simulink model "PubIfDecisionTOS_MDL"  (R2020b)
settings: configuration reference "DspaceConfig" (kept outside this file)
PostLoadFcn:
  | if any(exist('dsrtsu_mdlpostloadfcn', 'file') ~= 0), dsrtsu_mdlpostloadfcn('Execute', bdroot); end
InitFcn:
  | , if any(exist('dsmpb_private', 'file') ~= 0), dsmpb_private('dsmpb_mdlclblib', 'Init', bdroot); end,
undefined symbols (not defined in the file or in its folder): C_TOS_ACCEgoRAxletoFbumplength_m, C_TOS_ACCTargetFront_Flag, C_TOS_AEBJAPedObjDxThre_Val, C_TOS_AEBJAPedObjDyThre_Val, C_TOS_AEBJATargetSize_Val, C_TOS_AEBJAVehObjDxThre_Val, C_TOS_AEBJAVehObjDyThre_Val, C_TOS_AEBJuncPedTargetSize_Val, C_TOS_AEBLatObjDxThre_Val, C_TOS_AEBLatPedDyThre_Val, C_TOS_AEBLatTargetSize_Val, C_TOS_AEBLongTargetInEgoFront_Flag, C_TOS_axAbsGround_Parameter, C_TOS_CameraConfirmedFlag, C_TOS_CNsubjWidth, C_TOS_CurrentLaneCoreMinWidth_Val, C_TOS_CutInProb_Val_Zero, C_TOS_CutOutProb_Val_Zero, C_TOS_D2R_Val, C_TOS_DefaultValueObjectToCenterLine_dy, C_TOS_EgoCarWidth_Val, C_TOS_EgoDxRefPoint_m, C_TOS_EgoRAxletoFbumplength_m, C_TOS_HalfWidthVehicle_Con, C_TOS_HWA_CurrentLaneFlag, C_TOS_HWA_LeftLaneFlag, C_TOS_HWA_MovingDir_Vaild, C_TOS_HWA_MovState_Vaild, C_TOS_HWA_RightLaneFlag, C_TOS_LaneLineCourseErrorFront, C_TOS_LaneLineCourseErrorRear, C_TOS_MotorbikeDefaultWidth_m, C_TOS_NumberOfEffectiveTargets, C_TOS_Obj_Age_Val, C_TOS_Objdx_Constraint_Val, C_TOS_ObjectDefaultWidth_m, C_TOS_ObjInCurrentLane_Val, C_TOS_ObjInCurrentLaneValid, C_TOS_ObjInLeftLaneValid, C_TOS_ObjInRightLaneValid, C_TOS_ObjNotInCurrentLane_Val, C_TOS_ObjNotREElementType, C_TOS_ObjPredictDis_dy_ConstantVal_Zeros, C_TOS_ObjToCenterLine_ConstantVal_Zeros, C_TOS_OFMObjIDInvilad_Val, C_TOS_PIL_LatDisCons_Val_zero, C_TOS_PIL_ObjectCutInFlag_b, C_TOS_PIL_ObjectCutOutFlag_b, C_TOS_PIL_ObjLaneProb_al_Val, C_TOS_PP_ObjFusType_FC_Confirm_b, C_TOS_PP_ObjFusType_FC_FR_Confirm_b, C_TOS_PP_ObjFusType_FR_Confirm_b, C_TOS_RE_80BoolDefault_Val, C_TOS_RE_80Single181Default_Val, C_TOS_RE_80Single255Default_Val, C_TOS_RE_80Uint8Default_Val, C_TOS_RE_D2R, C_TOS_RE_D_180_Val, C_TOS_RE_InvalidObjectID_Val, C_TOS_RE_InvalidTargetChainDir_Val ... (+142)
libraries: simulink x1650, TOS_LIB x361, canfdmsglib x14
(part 38 of 69)

== system PubIfDecisionTOS_MDL/TOS_20201112/TOS_2012080320/TOS/AEB/TOS_AEBJunct_20201208/AEBJunc_Object_Condition1/AEBJA_TargetCondition/TOS_AEBJunc_TargetsCondition/AEBJunc_VehTargetCondition ==
  note: 过滤静止目标
  Object_ID : Inport
  PP_ObjFusType_FC_FR_Confirm : Inport  Port=2
  PP_ObjFusType_FR_Confirm : Inport  Port=3
  ObjectType : Inport  Port=4
  Object_Dx : Inport  Port=5
  Object_Dy : Inport  Port=6
  PP_ObjMovingDirSignalProcessing : Inport  Port=7
  Object_HeadingAngle : Inport  Port=8
  Object_VX : Inport  Port=9
  Object_VY : Inport  Port=10
  VIE_EgoVelocity : Inport  Port=11
  psiDtOpt : Inport  Port=12
  axvRefMs2 : Inport  Port=13
  AEBJunc_VehTarget_ObjectID_K1 : Inport  Port=14
  AEBJunc_Target_ObjectType_K1 : Inport  Port=15
  Object_MovingState : Inport  Port=16
  AEBJunc_VehTargetADxDyArea : Subsystem
  AEBJunc_VehTargetFusionTypeJudge : Subsystem
  AEBJunc_VehTargetObjectTypeFlag : Subsystem
  Chart : Stateflow chart  TreatAsAtomicUnit=on
  Compare To Constant : simulink/Logic and Bit Operations/Compare To Constant  relop===  const=true  OutDataTypeStr=boolean
  Logical Operator : Logic  Inputs=5  AllPortsSameDT=off  OutDataTypeStr=boolean
  Subsystem : Subsystem
  TOS_AEBJunc_VehTargetMoveDir : Subsystem
  Terminator : Terminator
  TOS_AEBJunc_VehTargetsDx : Outport
  AEBJunc_VehTargetFusionType_observal : Outport  Port=2
  AEBJunc_VehTargetObjectType_observal : Outport  Port=3
  AEBJunc_VehTargetDXDY_observal : Outport  Port=4
  AEBJunc_VehTargetMovDir_observal : Outport  Port=5
  AEBJunc_VehTargetMovState_observal : Outport  Port=6
  wires:
  [Object_ID] -> Chart/2(Object_ID)
  [AEBJunc_VehTarget_ObjectID_K1] -> Chart/4(AEBJunc_Target_ObjectID_K1)
  AEBJunc_VehTarget_ObjectID_K1/1 -> AEBJunc_VehTargetObjectTypeFlag/2(AEBJunc_VehTarget_ID_K1), [AEBJunc_VehTarget_ObjectID_K1]
  Object_ID/1 -> AEBJunc_VehTargetObjectTypeFlag/3(ObjectID), [Object_ID]
  [TOS_AEBJuncVehMovStateFlg] -> AEBJunc_VehTargetMovState_observal/1
  Subsystem/1(TOS_AEBJuncVehTargetMovStateFlg) -> [TOS_AEBJuncVehMovStateFlg], Logical Operator/5
  Object_MovingState/1 -> Subsystem/1(Object_MovingState)
  TOS_AEBJunc_VehTargetMoveDir/1(TOS_AEBJuncVehTargetMovDirFlg) -> [TOS_AEBJuncVehMovDirFlg], Logical Operator/4  "TOS_AEBJunc_VehTargetMovDir"
  Object_HeadingAngle/1 -> TOS_AEBJunc_VehTargetMoveDir/3(Object_HeadingAngle)
  PP_ObjFusType_FC_FR_Confirm/1 -> AEBJunc_VehTargetFusionTypeJudge/1(PP_ObjFusType_FC_FR_Confirm)
  [Object_Dx] -> TOS_AEBJunc_VehTargetMoveDir/1(Object_Dx)  "Object_Dx"
  [Object_Dx] -> Chart/6(Object_Dx)
  Object_Dx/1 -> [Object_Dx], AEBJunc_VehTargetADxDyArea/1(Object_Dx)
  [AEBJunc_VehFusionTypeFlag] -> AEBJunc_VehTargetFusionType_observal/1
  AEBJunc_VehTargetADxDyArea/1(TOS_AEBJunc_VehDxDyAreaFlag) -> Logical Operator/3, [TOS_AEBJunc_VehDxDyAreaFlag]
  Logical Operator/1 -> Compare To Constant/1
  Chart/1(TOS_AEBJunc_TargetsDx) -> TOS_AEBJunc_VehTargetsDx/1
  [AEBJunc_VehObjectTypeFlag] -> AEBJunc_VehTargetObjectType_observal/1
  PP_ObjMovingDirSignalProcessing/1 -> TOS_AEBJunc_VehTargetMoveDir/2(PP_ObjMovingDirSignalProcessing)
  psiDtOpt/1 -> Chart/3(psiDtOpt)
  PP_ObjFusType_FR_Confirm/1 -> AEBJunc_VehTargetFusionTypeJudge/2(PP_ObjFusType_FR_Confirm)
  Object_VY/1 -> [Object_Vy], TOS_AEBJunc_VehTargetMoveDir/5(Object_VY)
  VIE_EgoVelocity/1 -> TOS_AEBJunc_VehTargetMoveDir/6(VIE_EgoVelocity)
  AEBJunc_VehTargetFusionTypeJudge/1(AEBJunc_VehTargetFusionTypeFlag) -> [AEBJunc_VehFusionTypeFlag], Logical Operator/1
  Object_VX/1 -> TOS_AEBJunc_VehTargetMoveDir/4(Object_VX)
  Object_Dy/1 -> AEBJunc_VehTargetADxDyArea/2(Object_Dy)
  AEBJunc_VehTargetObjectTypeFlag/1(AEBJunc_VehTargetObjectTypeFlag) -> [AEBJunc_VehObjectTypeFlag], Logical Operator/2
  [TOS_AEBJuncVehMovDirFlg] -> AEBJunc_VehTargetMovDir_observal/1
  axvRefMs2/1 -> TOS_AEBJunc_VehTargetMoveDir/7(axvRefMs2)
  ObjectType/1 -> AEBJunc_VehTargetObjectTypeFlag/1(ObjectType)
  [TOS_AEBJunc_VehDxDyAreaFlag] -> AEBJunc_VehTargetDXDY_observal/1
  [Object_Vy] -> Chart/5(Object_Vy)
  Compare To Constant/1 -> Chart/1(AEBJunc_TargetCondition)
  AEBJunc_Target_ObjectType_K1/1 -> Terminator/1

== system PubIfDecisionTOS_MDL/TOS_20201112/TOS_2012080320/TOS/AEB/TOS_AEBLatCro1105/AEBLat_Object_Condition/AEBLat_TargetCondition/TOS_AEBLat_TargetsDx/AEBLat_TargetADxDyArea ==
  Object_Dx : Inport
  Object_Dy : Inport  Port=2
  Abs : Abs
  Compare To Constant1 : simulink/Logic and Bit Operations/Compare To Constant  relop=<=  const=C_TOS_AEBLatObjDxThre_Val  OutDataTypeStr=boolean
      settings: AttributesFormatString=C_TOS_AEBLatObjDxThre_Val = 40
  Compare To Constant2 : simulink/Logic and Bit Operations/Compare To Constant  relop=>  const=C_TOS_EgoDxRefPoint_m  OutDataTypeStr=boolean
      settings: AttributesFormatString=C_TOS_EgoDxRefPoint_m = 0
  Compare To Constant6 : simulink/Logic and Bit Operations/Compare To Constant  relop=<=  const=C_TOS_AEBLatPedDyThre_Val  OutDataTypeStr=boolean
      settings: AttributesFormatString=C_TOS_AEBLatPedDyThre_Val = 8 m
  Logical Operator : Logic  AllPortsSameDT=off  OutDataTypeStr=boolean
  Logical Operator1 : Logic  AllPortsSameDT=off  OutDataTypeStr=boolean
  TOS_AEBLat_DxDyAreaFlag : Outport
  wires:
  Logical Operator/1 -> Logical Operator1/1
  Object_Dy/1 -> Abs/1
  Abs/1 -> Compare To Constant6/1
  Compare To Constant1/1 -> Logical Operator/1
  Compare To Constant2/1 -> Logical Operator/2
  Logical Operator1/1 -> TOS_AEBLat_DxDyAreaFlag/1
  Compare To Constant6/1 -> Logical Operator1/2
  Object_Dx/1 -> Compare To Constant1/1, Compare To Constant2/1

== system PubIfDecisionTOS_MDL/TOS_20201112/TOS_2012080320/TOS/AEB/TOS_AEBLatCro1105/AEBLat_Object_Condition/AEBLat_TargetCondition/TOS_AEBLat_TargetsDx/AEBLat_TargetFusionTypeJudge ==
  PP_ObjFusType_FC_FR_Confirm : Inport
  PP_ObjFusType_FR_Confirm : Inport  Port=2
  Compare To Constant5 : simulink/Logic and Bit Operations/Compare To Constant  relop===  const=C_TOS_PP_ObjFusType_FC_FR_Confirm_b  OutDataTypeStr=boolean
      settings: AttributesFormatString=C_TOS_PP_ObjFusType_FC_FR_Confirm_b = 1
  Compare To Constant6 : simulink/Logic and Bit Operations/Compare To Constant  relop===  const=C_TOS_PP_ObjFusType_FR_Confirm_b  OutDataTypeStr=boolean
      settings: AttributesFormatString=C_TOS_PP_ObjFusType_FR_Confirm_b = 1
  Logical Operator : Logic  Operator=OR  AllPortsSameDT=off  OutDataTypeStr=boolean
  AEBLong_TargetFusionTypeFlag : Outport
  wires:
  PP_ObjFusType_FR_Confirm/1 -> Compare To Constant6/1
  PP_ObjFusType_FC_FR_Confirm/1 -> Compare To Constant5/1
  Compare To Constant6/1 -> Logical Operator/2
  Compare To Constant5/1 -> Logical Operator/1
  Logical Operator/1 -> AEBLong_TargetFusionTypeFlag/1

== system PubIfDecisionTOS_MDL/TOS_20201112/TOS_2012080320/TOS/AEB/TOS_AEBLatCro1105/AEBLat_Object_Condition/AEBLat_TargetCondition/TOS_AEBLat_TargetsDx/AEBLat_TargetObjectTypeFlag ==
  ObjectType : Inport
  AEBLat_Target_ID_K1 : Inport  Port=2
  ObjectID : Inport  Port=3
  AEBLat_TargetObjectTypeAborDly : Subsystem
  Compare To Constant3 : simulink/Logic and Bit Operations/Compare To Constant  relop===  const=OFM_OBJ_TYPE_E.PEDESTRIAN  OutDataTypeStr=boolean
      settings: AttributesFormatString=%<const>
  Compare To Constant4 : simulink/Logic and Bit Operations/Compare To Constant  relop===  const=OFM_OBJ_TYPE_E.MOTORBIKE  OutDataTypeStr=boolean
      settings: AttributesFormatString=%<const>
  Compare To Constant5 : simulink/Logic and Bit Operations/Compare To Constant  relop===  const=OFM_OBJ_TYPE_E.BICYCLE  OutDataTypeStr=boolean
      settings: AttributesFormatString=%<const>
  Data Type Conversion : DataTypeConversion  OutDataTypeStr=Enum: OFM_OBJ_TYPE_E
  Logical Operator3 : Logic  Operator=OR  Inputs=3  AllPortsSameDT=off  OutDataTypeStr=boolean
  AEBLat_TargetObjectTypeFlag : Outport
  wires:
  Data Type Conversion/1 -> Compare To Constant3/1, Compare To Constant4/1, Compare To Constant5/1
  ObjectType/1 -> Data Type Conversion/1
  Logical Operator3/1 -> AEBLat_TargetObjectTypeAborDly/3(TOS_AEBLat_ObjectType)
  Compare To Constant4/1 -> Logical Operator3/2
  Compare To Constant5/1 -> Logical Operator3/3
  Compare To Constant3/1 -> Logical Operator3/1
  ObjectID/1 -> AEBLat_TargetObjectTypeAborDly/2(ObjectID)
  AEBLat_Target_ID_K1/1 -> AEBLat_TargetObjectTypeAborDly/1(AEBLat_Target_ID_K1)
  AEBLat_TargetObjectTypeAborDly/1(TOS_AEBLatObjectTypeFilt) -> AEBLat_TargetObjectTypeFlag/1

== system PubIfDecisionTOS_MDL/TOS_20201112/TOS_2012080320/TOS/AEB/TOS_AEBLatCro1105/AEBLat_Object_Condition/AEBLat_TargetCondition/TOS_AEBLat_TargetsDx/TOS_AEBLat_TargetMoveDir ==
  Object_Dy : Inport
  PP_ObjMovingDirSignalProcessing : Inport  Port=2
  Object_HeadingAngle : Inport  Port=3
  Object_VX : Inport  Port=4
  Object_VY : Inport  Port=5
  VIE_EgoVelocity : Inport  Port=6
  Abs : Abs
  Abs1 : Abs
  Abs2 : Abs
  Add : Sum
  Compare To Constant : simulink/Logic and Bit Operations/Compare To Constant  relop=<  const=P_TOS_CrossingTarget_VxabsOffset_val  OutDataTypeStr=boolean
      settings: AttributesFormatString=%<const>
  Compare To Constant1 : simulink/Logic and Bit Operations/Compare To Constant  relop=>  const=P_TOS_CrossingTargetVyvThre_val  OutDataTypeStr=boolean
      settings: AttributesFormatString=%<const>
  Compare To Constant15 : simulink/Logic and Bit Operations/Compare To Constant  relop=>=  const=P_TOS_ObjLatCroYawAngMinThre_Val  OutDataTypeStr=boolean
      settings: AttributesFormatString=P_TOS_ObjLatCroYawAngMinThre_Val = 45
  Compare To Constant16 : simulink/Logic and Bit Operations/Compare To Constant  relop=<=  const=P_TOS_ObjLatCroYawAngMaxThre_Val  OutDataTypeStr=boolean
      settings: AttributesFormatString=P_TOS_ObjLatCroYawAngMaxThre_Val = 135
  Compare To Constant2 : simulink/Logic and Bit Operations/Compare To Constant  relop===  const=ObjectMovingOrientation_E.Crossing  OutDataTypeStr=boolean
      settings: AttributesFormatString=%<const>
  Data Type Conversion2 : DataTypeConversion  OutDataTypeStr=Enum: ObjectMovingOrientation_E
  Demux : Demux  Outputs=3
  Demux1 : Demux  Outputs=3
  Logical Operator : Logic  Operator=OR  Inputs=3  AllPortsSameDT=off  OutDataTypeStr=boolean
  Logical Operator{1..4,10} (5 alike) : Logic  AllPortsSameDT=off  OutDataTypeStr=boolean
  Logical Operator5 : Logic  Operator=OR  AllPortsSameDT=off  OutDataTypeStr=boolean
  Relational Operator : RelationalOperator  Operator=<  OutDataTypeStr=boolean  RndMeth=Simplest
  Relational Operator1 : RelationalOperator  Operator=<  OutDataTypeStr=boolean  RndMeth=Simplest
  Relational Operator2 : RelationalOperator  Operator=>  OutDataTypeStr=boolean  RndMeth=Simplest
  Relational Operator3 : RelationalOperator  Operator=>  OutDataTypeStr=boolean  RndMeth=Simplest
  Tapped Delay : simulink/Discrete/Tapped Delay  vinit=0.0  samptime=-1  NumDelays=2  DelayOrder=Oldest  includeCurrent=on
  TOS_AEBLatTargetMovDirFlg : Outport
  wires:
  Logical Operator/1 -> TOS_AEBLatTargetMovDirFlg/1
  PP_ObjMovingDirSignalProcessing/1 -> Data Type Conversion2/1
  Data Type Conversion2/1 -> Compare To Constant2/1
  Compare To Constant2/1 -> Logical Operator/1
  Object_HeadingAngle/1 -> Abs/1
  Abs/1 -> Compare To Constant16/1, Compare To Constant15/1
  Compare To Constant15/1 -> Logical Operator10/1
  Compare To Constant16/1 -> Logical Operator10/2
  Logical Operator10/1 -> Logical Operator/2
  Object_VX/1 -> Add/1
  VIE_EgoVelocity/1 -> Add/2
  Add/1 -> Abs1/1
  Abs1/1 -> Compare To Constant/1
  Compare To Constant/1 -> Logical Operator1/1
  Object_VY/1 -> Abs2/1
  Compare To Constant1/1 -> Logical Operator1/2
  Logical Operator1/1 -> Logical Operator2/1
  Object_Dy/1 -> Tapped Delay/1
  Demux/1 -> Relational Operator2/1
  Demux/2 -> Relational Operator3/1, Relational Operator2/2
  Demux/3 -> Relational Operator3/2
  Relational Operator2/1 -> Logical Operator3/1
  Relational Operator3/1 -> Logical Operator3/2
  Demux1/3 -> Relational Operator1/2
  Demux1/2 -> Relational Operator1/1, Relational Operator/2
  Demux1/1 -> Relational Operator/1
  Tapped Delay/1 -> Demux1/1, Demux/1
  Relational Operator/1 -> Logical Operator4/1
  Relational Operator1/1 -> Logical Operator4/2
  Logical Operator3/1 -> Logical Operator5/1
  Logical Operator4/1 -> Logical Operator5/2
  Logical Operator5/1 -> Logical Operator2/2
  Logical Operator2/1 -> Logical Operator/3
  Abs2/1 -> Compare To Constant1/1

== system PubIfDecisionTOS_MDL/TOS_20201112/TOS_2012080320/TOS/AEB/TOS_AEBLatCro1105/AEBLat_Object_Condition2/AEBLat_TargetCondition/TOS_AEBLat_TargetsDx/AEBLat_TargetADxDyArea ==
  Object_Dx : Inport
  Object_Dy : Inport  Port=2
  Abs : Abs
  Compare To Constant1 : simulink/Logic and Bit Operations/Compare To Constant  relop=<=  const=C_TOS_AEBLatObjDxThre_Val  OutDataTypeStr=boolean
      settings: AttributesFormatString=C_TOS_AEBLatObjDxThre_Val = 40
  Compare To Constant2 : simulink/Logic and Bit Operations/Compare To Constant  relop=>  const=C_TOS_EgoDxRefPoint_m  OutDataTypeStr=boolean
      settings: AttributesFormatString=C_TOS_EgoDxRefPoint_m = 0
  Compare To Constant6 : simulink/Logic and Bit Operations/Compare To Constant  relop=<=  const=C_TOS_AEBLatPedDyThre_Val  OutDataTypeStr=boolean
      settings: AttributesFormatString=C_TOS_AEBLatPedDyThre_Val = 8 m
  Logical Operator : Logic  AllPortsSameDT=off  OutDataTypeStr=boolean
  Logical Operator1 : Logic  AllPortsSameDT=off  OutDataTypeStr=boolean
  TOS_AEBLat_DxDyAreaFlag : Outport
  wires:
  Logical Operator/1 -> Logical Operator1/1
  Object_Dy/1 -> Abs/1
  Abs/1 -> Compare To Constant6/1
  Compare To Constant1/1 -> Logical Operator/1
  Compare To Constant2/1 -> Logical Operator/2
  Logical Operator1/1 -> TOS_AEBLat_DxDyAreaFlag/1
  Compare To Constant6/1 -> Logical Operator1/2
  Object_Dx/1 -> Compare To Constant1/1, Compare To Constant2/1

== system PubIfDecisionTOS_MDL/TOS_20201112/TOS_2012080320/TOS/AEB/TOS_AEBLatCro1105/AEBLat_Object_Condition2/AEBLat_TargetCondition/TOS_AEBLat_TargetsDx/AEBLat_TargetFusionTypeJudge ==
  PP_ObjFusType_FC_FR_Confirm : Inport
  PP_ObjFusType_FR_Confirm : Inport  Port=2
  Compare To Constant5 : simulink/Logic and Bit Operations/Compare To Constant  relop===  const=C_TOS_PP_ObjFusType_FC_FR_Confirm_b  OutDataTypeStr=boolean
      settings: AttributesFormatString=C_TOS_PP_ObjFusType_FC_FR_Confirm_b = 1
  Compare To Constant6 : simulink/Logic and Bit Operations/Compare To Constant  relop===  const=C_TOS_PP_ObjFusType_FR_Confirm_b  OutDataTypeStr=boolean
      settings: AttributesFormatString=C_TOS_PP_ObjFusType_FR_Confirm_b = 1
  Logical Operator : Logic  Operator=OR  AllPortsSameDT=off  OutDataTypeStr=boolean
  AEBLong_TargetFusionTypeFlag : Outport
  wires:
  PP_ObjFusType_FR_Confirm/1 -> Compare To Constant6/1
  PP_ObjFusType_FC_FR_Confirm/1 -> Compare To Constant5/1
  Compare To Constant6/1 -> Logical Operator/2
  Compare To Constant5/1 -> Logical Operator/1
  Logical Operator/1 -> AEBLong_TargetFusionTypeFlag/1

== system PubIfDecisionTOS_MDL/TOS_20201112/TOS_2012080320/TOS/AEB/TOS_AEBLatCro1105/AEBLat_Object_Condition2/AEBLat_TargetCondition/TOS_AEBLat_TargetsDx/AEBLat_TargetObjectTypeFlag ==
  ObjectType : Inport
  Compare To Constant3 : simulink/Logic and Bit Operations/Compare To Constant  relop===  const=OFM_OBJ_TYPE_E.PEDESTRIAN  OutDataTypeStr=boolean
      settings: AttributesFormatString=%<const>
  Compare To Constant4 : simulink/Logic and Bit Operations/Compare To Constant  relop===  const=OFM_OBJ_TYPE_E.MOTORBIKE  OutDataTypeStr=boolean
      settings: AttributesFormatString=%<const>
  Compare To Constant5 : simulink/Logic and Bit Operations/Compare To Constant  relop===  const=OFM_OBJ_TYPE_E.BICYCLE  OutDataTypeStr=boolean
      settings: AttributesFormatString=%<const>
  Data Type Conversion : DataTypeConversion  OutDataTypeStr=Enum: OFM_OBJ_TYPE_E
  Logical Operator3 : Logic  Operator=OR  Inputs=3  AllPortsSameDT=off  OutDataTypeStr=boolean
  AEBLat_TargetObjectTypeFlag : Outport
  wires:
  Data Type Conversion/1 -> Compare To Constant3/1, Compare To Constant5/1, Compare To Constant4/1
  Compare To Constant5/1 -> Logical Operator3/3
  ObjectType/1 -> Data Type Conversion/1
  Compare To Constant4/1 -> Logical Operator3/2
  Compare To Constant3/1 -> Logical Operator3/1
  Logical Operator3/1 -> AEBLat_TargetObjectTypeFlag/1

== system PubIfDecisionTOS_MDL/TOS_20201112/TOS_2012080320/TOS/AEB/TOS_AEBLatCro1105/AEBLat_Object_Condition2/AEBLat_TargetCondition/TOS_AEBLat_TargetsDx/TOS_AEBLat_TargetMoveDir ==
  Object_Dy : Inport
  PP_ObjMovingDirSignalProcessing : Inport  Port=2
  Object_HeadingAngle : Inport  Port=3
  Object_VX : Inport  Port=4
  Object_VY : Inport  Port=5
  VIE_EgoVelocity : Inport  Port=6
  Abs : Abs
  Abs1 : Abs
  Abs2 : Abs
  Add : Sum
  Compare To Constant : simulink/Logic and Bit Operations/Compare To Constant  relop=<  const=P_TOS_CrossingTarget_VxabsOffset_val  OutDataTypeStr=boolean
      settings: AttributesFormatString=%<const>
  Compare To Constant1 : simulink/Logic and Bit Operations/Compare To Constant  relop=>  const=P_TOS_CrossingTargetVyvThre_val  OutDataTypeStr=boolean
      settings: AttributesFormatString=%<const>
  Compare To Constant15 : simulink/Logic and Bit Operations/Compare To Constant  relop=>=  const=P_TOS_ObjLatCroYawAngMinThre_Val  OutDataTypeStr=boolean
      settings: AttributesFormatString=P_TOS_ObjLatCroYawAngMinThre_Val = 45
  Compare To Constant16 : simulink/Logic and Bit Operations/Compare To Constant  relop=<=  const=P_TOS_ObjLatCroYawAngMaxThre_Val  OutDataTypeStr=boolean
      settings: AttributesFormatString=P_TOS_ObjLatCroYawAngMaxThre_Val = 135
  Compare To Constant2 : simulink/Logic and Bit Operations/Compare To Constant  relop===  const=ObjectMovingOrientation_E.Crossing  OutDataTypeStr=boolean
      settings: AttributesFormatString=%<const>
  Data Type Conversion2 : DataTypeConversion  OutDataTypeStr=Enum: ObjectMovingOrientation_E
  Demux : Demux  Outputs=3
  Demux1 : Demux  Outputs=3
  Logical Operator : Logic  Operator=OR  Inputs=3  AllPortsSameDT=off  OutDataTypeStr=boolean
  Logical Operator{1..4,10} (5 alike) : Logic  AllPortsSameDT=off  OutDataTypeStr=boolean
  Logical Operator5 : Logic  Operator=OR  AllPortsSameDT=off  OutDataTypeStr=boolean
  Relational Operator : RelationalOperator  Operator=<  OutDataTypeStr=boolean  RndMeth=Simplest
  Relational Operator1 : RelationalOperator  Operator=<  OutDataTypeStr=boolean  RndMeth=Simplest
  Relational Operator2 : RelationalOperator  Operator=>  OutDataTypeStr=boolean  RndMeth=Simplest
  Relational Operator3 : RelationalOperator  Operator=>  OutDataTypeStr=boolean  RndMeth=Simplest
  Tapped Delay : simulink/Discrete/Tapped Delay  vinit=0.0  samptime=-1  NumDelays=2  DelayOrder=Oldest  includeCurrent=on
  TOS_AEBLatTargetMovDirFlg : Outport
  wires:
  Logical Operator/1 -> TOS_AEBLatTargetMovDirFlg/1
  PP_ObjMovingDirSignalProcessing/1 -> Data Type Conversion2/1
  Data Type Conversion2/1 -> Compare To Constant2/1
  Compare To Constant2/1 -> Logical Operator/1
  Object_HeadingAngle/1 -> Abs/1
  Abs/1 -> Compare To Constant16/1, Compare To Constant15/1
  Compare To Constant15/1 -> Logical Operator10/1
  Compare To Constant16/1 -> Logical Operator10/2
  Logical Operator10/1 -> Logical Operator/2
  Object_VX/1 -> Add/1
  VIE_EgoVelocity/1 -> Add/2
  Add/1 -> Abs1/1
  Abs1/1 -> Compare To Constant/1
  Compare To Constant/1 -> Logical Operator1/1
  Object_VY/1 -> Abs2/1
  Compare To Constant1/1 -> Logical Operator1/2
  Logical Operator1/1 -> Logical Operator2/1
  Object_Dy/1 -> Tapped Delay/1
  Demux/1 -> Relational Operator2/1
  Demux/2 -> Relational Operator3/1, Relational Operator2/2
  Demux/3 -> Relational Operator3/2
  Relational Operator2/1 -> Logical Operator3/1
  Relational Operator3/1 -> Logical Operator3/2
  Demux1/3 -> Relational Operator1/2
  Demux1/2 -> Relational Operator1/1, Relational Operator/2
  Demux1/1 -> Relational Operator/1
  Tapped Delay/1 -> Demux1/1, Demux/1
  Relational Operator/1 -> Logical Operator4/1
  Relational Operator1/1 -> Logical Operator4/2
  Logical Operator3/1 -> Logical Operator5/1
  Logical Operator4/1 -> Logical Operator5/2
  Logical Operator5/1 -> Logical Operator2/2
  Logical Operator2/1 -> Logical Operator/3
  Abs2/1 -> Compare To Constant1/1

== system PubIfDecisionTOS_MDL/TOS_20201112/TOS_2012080320/TOS/AEB/TOS_AEBLatCro_20201208/AEBLat_Object_Condition/AEBLat_TargetCondition/TOS_AEBLat_TargetsDx/AEBLat_TargetADxDyArea ==
  Object_Dx : Inport
  Object_Dy : Inport  Port=2
  Abs : Abs
  Compare To Constant1 : simulink/Logic and Bit Operations/Compare To Constant  relop=<=  const=C_TOS_AEBLatObjDxThre_Val  OutDataTypeStr=boolean
      settings: AttributesFormatString=C_TOS_AEBLatObjDxThre_Val = 40
  Compare To Constant2 : simulink/Logic and Bit Operations/Compare To Constant  relop=>  const=C_TOS_EgoDxRefPoint_m  OutDataTypeStr=boolean
      settings: AttributesFormatString=C_TOS_EgoDxRefPoint_m = 0
  Compare To Constant6 : simulink/Logic and Bit Operations/Compare To Constant  relop=<=  const=C_TOS_AEBLatPedDyThre_Val  OutDataTypeStr=boolean
      settings: AttributesFormatString=C_TOS_AEBLatPedDyThre_Val = 8 m
  Logical Operator : Logic  AllPortsSameDT=off  OutDataTypeStr=boolean
  Logical Operator1 : Logic  AllPortsSameDT=off  OutDataTypeStr=boolean
  TOS_AEBLat_DxDyAreaFlag : Outport
  wires:
  Logical Operator/1 -> Logical Operator1/1
  Object_Dy/1 -> Abs/1
  Abs/1 -> Compare To Constant6/1
  Compare To Constant1/1 -> Logical Operator/1
  Compare To Constant2/1 -> Logical Operator/2
  Logical Operator1/1 -> TOS_AEBLat_DxDyAreaFlag/1
  Compare To Constant6/1 -> Logical Operator1/2
  Object_Dx/1 -> Compare To Constant1/1, Compare To Constant2/1

== system PubIfDecisionTOS_MDL/TOS_20201112/TOS_2012080320/TOS/AEB/TOS_AEBLatCro_20201208/AEBLat_Object_Condition/AEBLat_TargetCondition/TOS_AEBLat_TargetsDx/AEBLat_TargetFusionTypeJudge ==
  PP_ObjFusType_FC_FR_Confirm : Inport
  PP_ObjFusType_FR_Confirm : Inport  Port=2
  Compare To Constant5 : simulink/Logic and Bit Operations/Compare To Constant  relop===  const=C_TOS_PP_ObjFusType_FC_FR_Confirm_b  OutDataTypeStr=boolean
      settings: AttributesFormatString=C_TOS_PP_ObjFusType_FC_FR_Confirm_b = 1
  Compare To Constant6 : simulink/Logic and Bit Operations/Compare To Constant  relop===  const=C_TOS_PP_ObjFusType_FR_Confirm_b  OutDataTypeStr=boolean
      settings: AttributesFormatString=C_TOS_PP_ObjFusType_FR_Confirm_b = 1
  Logical Operator : Logic  Operator=OR  AllPortsSameDT=off  OutDataTypeStr=boolean
  AEBLong_TargetFusionTypeFlag : Outport
  wires:
  PP_ObjFusType_FR_Confirm/1 -> Compare To Constant6/1
  PP_ObjFusType_FC_FR_Confirm/1 -> Compare To Constant5/1
  Compare To Constant6/1 -> Logical Operator/2
  Compare To Constant5/1 -> Logical Operator/1
  Logical Operator/1 -> AEBLong_TargetFusionTypeFlag/1

== system PubIfDecisionTOS_MDL/TOS_20201112/TOS_2012080320/TOS/AEB/TOS_AEBLatCro_20201208/AEBLat_Object_Condition/AEBLat_TargetCondition/TOS_AEBLat_TargetsDx/AEBLat_TargetObjectTypeFlag ==
  ObjectType : Inport
  AEBLat_Target_ID_K1 : Inport  Port=2
  ObjectID : Inport  Port=3
  AEBLat_TargetObjectTypeAborDly : Subsystem
  Compare To Constant3 : simulink/Logic and Bit Operations/Compare To Constant  relop===  const=OFM_OBJ_TYPE_E.PEDESTRIAN  OutDataTypeStr=boolean
      settings: AttributesFormatString=%<const>
  Compare To Constant4 : simulink/Logic and Bit Operations/Compare To Constant  relop===  const=OFM_OBJ_TYPE_E.MOTORBIKE  OutDataTypeStr=boolean
      settings: AttributesFormatString=%<const>
  Compare To Constant5 : simulink/Logic and Bit Operations/Compare To Constant  relop===  const=OFM_OBJ_TYPE_E.BICYCLE  OutDataTypeStr=boolean
      settings: AttributesFormatString=%<const>
  Data Type Conversion : DataTypeConversion  OutDataTypeStr=Enum: OFM_OBJ_TYPE_E
  Logical Operator3 : Logic  Operator=OR  Inputs=3  AllPortsSameDT=off  OutDataTypeStr=boolean
  AEBLat_TargetObjectTypeFlag : Outport
  wires:
  Data Type Conversion/1 -> Compare To Constant3/1, Compare To Constant4/1, Compare To Constant5/1
  ObjectType/1 -> Data Type Conversion/1
  Logical Operator3/1 -> AEBLat_TargetObjectTypeAborDly/3(TOS_AEBLat_ObjectType)
  Compare To Constant4/1 -> Logical Operator3/2
  Compare To Constant5/1 -> Logical Operator3/3
  Compare To Constant3/1 -> Logical Operator3/1
  ObjectID/1 -> AEBLat_TargetObjectTypeAborDly/2(ObjectID)
  AEBLat_Target_ID_K1/1 -> AEBLat_TargetObjectTypeAborDly/1(AEBLat_Target_ID_K1)
  AEBLat_TargetObjectTypeAborDly/1(TOS_AEBLatObjectTypeFilt) -> AEBLat_TargetObjectTypeFlag/1

== system PubIfDecisionTOS_MDL/TOS_20201112/TOS_2012080320/TOS/AEB/TOS_AEBLatCro_20201208/AEBLat_Object_Condition/AEBLat_TargetCondition/TOS_AEBLat_TargetsDx/TOS_AEBLat_TargetMoveDir ==
  Object_Dy : Inport
  PP_ObjMovingDirSignalProcessing : Inport  Port=2
  Object_HeadingAngle : Inport  Port=3
  Object_VX : Inport  Port=4
  Object_VY : Inport  Port=5
  VIE_EgoVelocity : Inport  Port=6
  AEBLat_Target_ID_K1 : Inport  Port=7
  ObjectID : Inport  Port=8
  AEBLat_TargetMovDirAborDly : Subsystem
  Abs : Abs
  Abs1 : Abs
  Abs2 : Abs
  Add : Sum
  Compare To Constant : simulink/Logic and Bit Operations/Compare To Constant  relop=<  const=P_TOS_CrossingTarget_VxabsOffset_val  OutDataTypeStr=boolean
      settings: AttributesFormatString=%<const>
  Compare To Constant1 : simulink/Logic and Bit Operations/Compare To Constant  relop=>  const=P_TOS_CrossingTargetVyvThre_val  OutDataTypeStr=boolean
      settings: AttributesFormatString=%<const>
  Compare To Constant15 : simulink/Logic and Bit Operations/Compare To Constant  relop=>=  const=P_TOS_ObjLatCroYawAngMinThre_Val  OutDataTypeStr=boolean
      settings: AttributesFormatString=P_TOS_ObjLatCroYawAngMinThre_Val = 45
  Compare To Constant16 : simulink/Logic and Bit Operations/Compare To Constant  relop=<=  const=P_TOS_ObjLatCroYawAngMaxThre_Val  OutDataTypeStr=boolean
      settings: AttributesFormatString=P_TOS_ObjLatCroYawAngMaxThre_Val = 135
  Compare To Constant2 : simulink/Logic and Bit Operations/Compare To Constant  relop===  const=ObjectMovingOrientation_E.Crossing  OutDataTypeStr=boolean
      settings: AttributesFormatString=%<const>
  Data Type Conversion2 : DataTypeConversion  OutDataTypeStr=Enum: ObjectMovingOrientation_E
  Demux : Demux  Outputs=3
  Demux1 : Demux  Outputs=3
  Logical Operator : Logic  Operator=OR  Inputs=3  AllPortsSameDT=off  OutDataTypeStr=boolean
  Logical Operator{1..4,10} (5 alike) : Logic  AllPortsSameDT=off  OutDataTypeStr=boolean
  Logical Operator5 : Logic  Operator=OR  AllPortsSameDT=off  OutDataTypeStr=boolean
  Relational Operator : RelationalOperator  Operator=<  OutDataTypeStr=boolean  RndMeth=Simplest
  Relational Operator1 : RelationalOperator  Operator=<  OutDataTypeStr=boolean  RndMeth=Simplest
  Relational Operator2 : RelationalOperator  Operator=>  OutDataTypeStr=boolean  RndMeth=Simplest
  Relational Operator3 : RelationalOperator  Operator=>  OutDataTypeStr=boolean  RndMeth=Simplest
  Tapped Delay : simulink/Discrete/Tapped Delay  vinit=0.0  samptime=-1  NumDelays=2  DelayOrder=Oldest  includeCurrent=on
  TOS_AEBLatTargetMovDirFlg : Outport
  wires:
  Logical Operator/1 -> AEBLat_TargetMovDirAborDly/3(TOS_AEBLat_MovDir_Flag)
  PP_ObjMovingDirSignalProcessing/1 -> Data Type Conversion2/1
  Data Type Conversion2/1 -> Compare To Constant2/1
  Compare To Constant2/1 -> Logical Operator/1
  Object_HeadingAngle/1 -> Abs/1
  Abs/1 -> Compare To Constant16/1, Compare To Constant15/1
  Compare To Constant15/1 -> Logical Operator10/1
  Compare To Constant16/1 -> Logical Operator10/2
  Logical Operator10/1 -> Logical Operator/2
  Object_VX/1 -> Add/1
  VIE_EgoVelocity/1 -> Add/2
  Add/1 -> Abs1/1
  Abs1/1 -> Compare To Constant/1
  Compare To Constant/1 -> Logical Operator1/1
  Object_VY/1 -> Abs2/1
  Compare To Constant1/1 -> Logical Operator1/2
  Logical Operator1/1 -> Logical Operator2/1
  Object_Dy/1 -> Tapped Delay/1
  Demux/1 -> Relational Operator2/1
  Demux/2 -> Relational Operator3/1, Relational Operator2/2
  Demux/3 -> Relational Operator3/2
  Relational Operator2/1 -> Logical Operator3/1
  Relational Operator3/1 -> Logical Operator3/2
  Demux1/3 -> Relational Operator1/2
  Demux1/2 -> Relational Operator1/1, Relational Operator/2
  Demux1/1 -> Relational Operator/1
  Tapped Delay/1 -> Demux1/1, Demux/1
  Relational Operator/1 -> Logical Operator4/1
  Relational Operator1/1 -> Logical Operator4/2
  Logical Operator3/1 -> Logical Operator5/1
  Logical Operator4/1 -> Logical Operator5/2
  Logical Operator5/1 -> Logical Operator2/2
  Logical Operator2/1 -> Logical Operator/3
  Abs2/1 -> Compare To Constant1/1
  ObjectID/1 -> AEBLat_TargetMovDirAborDly/2(ObjectID)
  AEBLat_Target_ID_K1/1 -> AEBLat_TargetMovDirAborDly/1(AEBLat_Target_ID_K1)
  AEBLat_TargetMovDirAborDly/1(TOS_AEBLat_MovDirFlag_Delay) -> TOS_AEBLatTargetMovDirFlg/1

== system PubIfDecisionTOS_MDL/TOS_20201112/TOS_2012080320/TOS/AEB/TOS_AEBLatCro_20201208/AEBLat_Object_Condition2/AEBLat_TargetCondition/TOS_AEBLat_TargetsDx/AEBLat_TargetADxDyArea ==
  Object_Dx : Inport
  Object_Dy : Inport  Port=2
  Abs : Abs
  Compare To Constant1 : simulink/Logic and Bit Operations/Compare To Constant  relop=<=  const=C_TOS_AEBLatObjDxThre_Val  OutDataTypeStr=boolean
      settings: AttributesFormatString=C_TOS_AEBLatObjDxThre_Val = 40
  Compare To Constant2 : simulink/Logic and Bit Operations/Compare To Constant  relop=>  const=C_TOS_EgoDxRefPoint_m  OutDataTypeStr=boolean
      settings: AttributesFormatString=C_TOS_EgoDxRefPoint_m = 0
  Compare To Constant6 : simulink/Logic and Bit Operations/Compare To Constant  relop=<=  const=C_TOS_AEBLatPedDyThre_Val  OutDataTypeStr=boolean
      settings: AttributesFormatString=C_TOS_AEBLatPedDyThre_Val = 8 m
  Logical Operator : Logic  AllPortsSameDT=off  OutDataTypeStr=boolean
  Logical Operator1 : Logic  AllPortsSameDT=off  OutDataTypeStr=boolean
  TOS_AEBLat_DxDyAreaFlag : Outport
  wires:
  Logical Operator/1 -> Logical Operator1/1
  Object_Dy/1 -> Abs/1
  Abs/1 -> Compare To Constant6/1
  Compare To Constant1/1 -> Logical Operator/1
  Compare To Constant2/1 -> Logical Operator/2
  Logical Operator1/1 -> TOS_AEBLat_DxDyAreaFlag/1
  Compare To Constant6/1 -> Logical Operator1/2
  Object_Dx/1 -> Compare To Constant1/1, Compare To Constant2/1

== system PubIfDecisionTOS_MDL/TOS_20201112/TOS_2012080320/TOS/AEB/TOS_AEBLatCro_20201208/AEBLat_Object_Condition2/AEBLat_TargetCondition/TOS_AEBLat_TargetsDx/AEBLat_TargetFusionTypeJudge ==
  PP_ObjFusType_FC_FR_Confirm : Inport
  PP_ObjFusType_FR_Confirm : Inport  Port=2
  Compare To Constant5 : simulink/Logic and Bit Operations/Compare To Constant  relop===  const=C_TOS_PP_ObjFusType_FC_FR_Confirm_b  OutDataTypeStr=boolean
      settings: AttributesFormatString=C_TOS_PP_ObjFusType_FC_FR_Confirm_b = 1
  Compare To Constant6 : simulink/Logic and Bit Operations/Compare To Constant  relop===  const=C_TOS_PP_ObjFusType_FR_Confirm_b  OutDataTypeStr=boolean
      settings: AttributesFormatString=C_TOS_PP_ObjFusType_FR_Confirm_b = 1
  Logical Operator : Logic  Operator=OR  AllPortsSameDT=off  OutDataTypeStr=boolean
  AEBLong_TargetFusionTypeFlag : Outport
  wires:
  PP_ObjFusType_FR_Confirm/1 -> Compare To Constant6/1
  PP_ObjFusType_FC_FR_Confirm/1 -> Compare To Constant5/1
  Compare To Constant6/1 -> Logical Operator/2
  Compare To Constant5/1 -> Logical Operator/1
  Logical Operator/1 -> AEBLong_TargetFusionTypeFlag/1

== system PubIfDecisionTOS_MDL/TOS_20201112/TOS_2012080320/TOS/AEB/TOS_AEBLatCro_20201208/AEBLat_Object_Condition2/AEBLat_TargetCondition/TOS_AEBLat_TargetsDx/AEBLat_TargetObjectTypeFlag ==
  ObjectType : Inport
  Compare To Constant3 : simulink/Logic and Bit Operations/Compare To Constant  relop===  const=OFM_OBJ_TYPE_E.PEDESTRIAN  OutDataTypeStr=boolean
      settings: AttributesFormatString=%<const>
  Compare To Constant4 : simulink/Logic and Bit Operations/Compare To Constant  relop===  const=OFM_OBJ_TYPE_E.MOTORBIKE  OutDataTypeStr=boolean
      settings: AttributesFormatString=%<const>
  Compare To Constant5 : simulink/Logic and Bit Operations/Compare To Constant  relop===  const=OFM_OBJ_TYPE_E.BICYCLE  OutDataTypeStr=boolean
      settings: AttributesFormatString=%<const>
  Data Type Conversion : DataTypeConversion  OutDataTypeStr=Enum: OFM_OBJ_TYPE_E
  Logical Operator3 : Logic  Operator=OR  Inputs=3  AllPortsSameDT=off  OutDataTypeStr=boolean
  AEBLat_TargetObjectTypeFlag : Outport
  wires:
  Data Type Conversion/1 -> Compare To Constant3/1, Compare To Constant5/1, Compare To Constant4/1
  Compare To Constant5/1 -> Logical Operator3/3
  ObjectType/1 -> Data Type Conversion/1
  Compare To Constant4/1 -> Logical Operator3/2
  Compare To Constant3/1 -> Logical Operator3/1
  Logical Operator3/1 -> AEBLat_TargetObjectTypeFlag/1

== system PubIfDecisionTOS_MDL/TOS_20201112/TOS_2012080320/TOS/AEB/TOS_AEBLatCro_20201208/AEBLat_Object_Condition2/AEBLat_TargetCondition/TOS_AEBLat_TargetsDx/TOS_AEBLat_TargetMoveDir ==
  Object_Dy : Inport
  PP_ObjMovingDirSignalProcessing : Inport  Port=2
  Object_HeadingAngle : Inport  Port=3
  Object_VX : Inport  Port=4
  Object_VY : Inport  Port=5
  VIE_EgoVelocity : Inport  Port=6
  Abs : Abs
  Abs1 : Abs
  Abs2 : Abs
  Add : Sum
  Compare To Constant : simulink/Logic and Bit Operations/Compare To Constant  relop=<  const=P_TOS_CrossingTarget_VxabsOffset_val  OutDataTypeStr=boolean
      settings: AttributesFormatString=%<const>
  Compare To Constant1 : simulink/Logic and Bit Operations/Compare To Constant  relop=>  const=P_TOS_CrossingTargetVyvThre_val  OutDataTypeStr=boolean
      settings: AttributesFormatString=%<const>
  Compare To Constant15 : simulink/Logic and Bit Operations/Compare To Constant  relop=>=  const=P_TOS_ObjLatCroYawAngMinThre_Val  OutDataTypeStr=boolean
      settings: AttributesFormatString=P_TOS_ObjLatCroYawAngMinThre_Val = 45
  Compare To Constant16 : simulink/Logic and Bit Operations/Compare To Constant  relop=<=  const=P_TOS_ObjLatCroYawAngMaxThre_Val  OutDataTypeStr=boolean
      settings: AttributesFormatString=P_TOS_ObjLatCroYawAngMaxThre_Val = 135
  Compare To Constant2 : simulink/Logic and Bit Operations/Compare To Constant  relop===  const=ObjectMovingOrientation_E.Crossing  OutDataTypeStr=boolean
      settings: AttributesFormatString=%<const>
  Data Type Conversion2 : DataTypeConversion  OutDataTypeStr=Enum: ObjectMovingOrientation_E
  Demux : Demux  Outputs=3
  Demux1 : Demux  Outputs=3
  Logical Operator : Logic  Operator=OR  Inputs=3  AllPortsSameDT=off  OutDataTypeStr=boolean
  Logical Operator{1..4,10} (5 alike) : Logic  AllPortsSameDT=off  OutDataTypeStr=boolean
  Logical Operator5 : Logic  Operator=OR  AllPortsSameDT=off  OutDataTypeStr=boolean
  Relational Operator : RelationalOperator  Operator=<  OutDataTypeStr=boolean  RndMeth=Simplest
  Relational Operator1 : RelationalOperator  Operator=<  OutDataTypeStr=boolean  RndMeth=Simplest
  Relational Operator2 : RelationalOperator  Operator=>  OutDataTypeStr=boolean  RndMeth=Simplest
  Relational Operator3 : RelationalOperator  Operator=>  OutDataTypeStr=boolean  RndMeth=Simplest
  Tapped Delay : simulink/Discrete/Tapped Delay  vinit=0.0  samptime=-1  NumDelays=2  DelayOrder=Oldest  includeCurrent=on
  TOS_AEBLatTargetMovDirFlg : Outport
  wires:
  Logical Operator/1 -> TOS_AEBLatTargetMovDirFlg/1
  PP_ObjMovingDirSignalProcessing/1 -> Data Type Conversion2/1
  Data Type Conversion2/1 -> Compare To Constant2/1
  Compare To Constant2/1 -> Logical Operator/1
  Object_HeadingAngle/1 -> Abs/1
  Abs/1 -> Compare To Constant16/1, Compare To Constant15/1
  Compare To Constant15/1 -> Logical Operator10/1
  Compare To Constant16/1 -> Logical Operator10/2
  Logical Operator10/1 -> Logical Operator/2
  Object_VX/1 -> Add/1
  VIE_EgoVelocity/1 -> Add/2
  Add/1 -> Abs1/1
  Abs1/1 -> Compare To Constant/1
  Compare To Constant/1 -> Logical Operator1/1
  Object_VY/1 -> Abs2/1
  Compare To Constant1/1 -> Logical Operator1/2
  Logical Operator1/1 -> Logical Operator2/1
  Object_Dy/1 -> Tapped Delay/1
  Demux/1 -> Relational Operator2/1
  Demux/2 -> Relational Operator3/1, Relational Operator2/2
  Demux/3 -> Relational Operator3/2
  Relational Operator2/1 -> Logical Operator3/1
  Relational Operator3/1 -> Logical Operator3/2
  Demux1/3 -> Relational Operator1/2
  Demux1/2 -> Relational Operator1/1, Relational Operator/2
  Demux1/1 -> Relational Operator/1
  Tapped Delay/1 -> Demux1/1, Demux/1
  Relational Operator/1 -> Logical Operator4/1
  Relational Operator1/1 -> Logical Operator4/2
  Logical Operator3/1 -> Logical Operator5/1
  Logical Operator4/1 -> Logical Operator5/2
  Logical Operator5/1 -> Logical Operator2/2
  Logical Operator2/1 -> Logical Operator/3
  Abs2/1 -> Compare To Constant1/1

== system PubIfDecisionTOS_MDL/TOS_20201112/TOS_2012080320/TOS/AEB/TOS_AEBLong/AEBLongTargetInfor/AEBLongTargetMovingDir/AEBLongTargetMovingDir/Subsystem ==
  PP_MovingState : Inport
  AEBLongTargetIndex : Inport  Port=2
  PP_MovingDir : Inport  Port=3
  Compare To Constant : simulink/Logic and Bit Operations/Compare To Constant  relop===  const=ObjectMovingState_AEB_E.Still  OutDataTypeStr=boolean
  Data Type Conversion : DataTypeConversion  OutDataTypeStr=Enum: ObjectMovingState_AEB_E
  Data Type Conversion1 : DataTypeConversion  OutDataTypeStr=Enum: ObjectMovingOrientation_E
  Data Type Conversion2 : DataTypeConversion  OutDataTypeStr=uint8
  Enumerated Constant : simulink/Sources/Enumerated Constant  OutDataTypeStr=Enum: ObjectMovingOrientation_E  Value=ObjectMovingOrientation_E.SameDir  SampleTime=inf
  Selector : Selector  InputPortWidth=80  IndexOptions=Index vector (port)  Indices=[1 3]  OutputSizes=1
  Selector1 : Selector  InputPortWidth=80  IndexOptions=Index vector (port)  Indices=[1 3]  OutputSizes=1
  Switch : Switch  Criteria=u2 ~= 0
  TOS_AEBLongTargetMovingDir : Outport
  wires:
  Data Type Conversion1/1 -> Switch/3
  Enumerated Constant/1 -> Switch/1
  Data Type Conversion/1 -> Compare To Constant/1
  Switch/1 -> Data Type Conversion2/1
  Selector1/1 -> Data Type Conversion1/1
  Selector/1 -> Data Type Conversion/1
  Compare To Constant/1 -> Switch/2
  Data Type Conversion2/1 -> TOS_AEBLongTargetMovingDir/1
  PP_MovingState/1 -> Selector/1
  PP_MovingDir/1 -> Selector1/1
  AEBLongTargetIndex/1 -> Selector1/2, Selector/2
